simulink model "processo_fig_7_7_b_NISE1"  (R2017b)
settings: Solver=VariableStepAuto  StartTime=0.0  StopTime=3  RelTol=1e-3
settings Model: Creator=fernandopassold  LastModifiedBy=fernandopassold
settings CodeAppCC: StateflowObjectComments=on

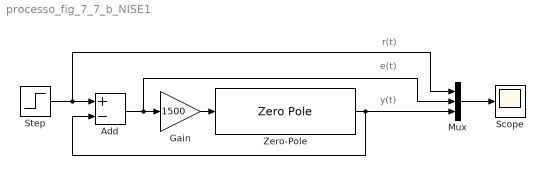
== system processo_fig_7_7_b_NISE1 ==
  note: y(t)
  note: e(t)
  note: r(t)
  Add : Sum  Inputs=+-
  Gain : Gain  Gain=1500
  Mux : Mux  Inputs=3
  Scope : Scope
  Step : Step  SampleTime=0
  Zero-Pole : ZeroPole  Zeros=[-2 -5 -6]  Poles=[0 -8 -10 -12]
  wires:
  Mux/1 -> Scope/1
  Add/1 -> Mux/2, Gain/1
  Step/1 -> Mux/1, Add/1
  Gain/1 -> Zero-Pole/1
  Zero-Pole/1 -> Mux/3, Add/2
